simulink model "FishEyeTestNonCardboard_cs_old"  (R2018b)
settings: Solver=ode5  StartTime=0.0  StopTime=40  FixedStep=1/20  RelTol=1e-3
PreLoadFcn:
  | mbxruntime.callbacks.PreLoadFcn(bdroot);
PostLoadFcn:
  | mbxruntime.callbacks.PostLoadFcn(bdroot);
InitFcn:
  | mbxruntime.callbacks.InitFcn(bdroot);
StartFcn:
  | mbxruntime.callbacks.StartFcn(bdroot);
StopFcn:
  | mbxruntime.callbacks.StopFcn(bdroot);
model workspace (MAT data in the model file):
  mbox_table : struct (value not decoded)
  model_closed = 0
  sim_status = 0
undefined symbols (not defined in the file or in its folder): InitImageOutputDir
libraries: PreScanSimulinkLibrary x6, instrumentlib x1, simulink_extras x1
(part 1 of 2)
CloseFcn:
  | mbxruntime.callbacks.CloseFcn(bdroot);
settings Model: Creator=PRESCAN  LastModifiedBy=Kimoss
settings DataIOCC: LimitDataPoints=on  SaveFormat=Array  SignalLoggingSaveFormat=ModelDataLogs
settings OptimizationCC: ExpressionDepthLimit=2147483647  InitFltsAndDblsToZero=on  LifeSpan=inf
settings DebuggingCC: SaveWithParameterizedLinksMsg=none  UnderspecifiedInitializationDetection=Classic  MergeDetectMultiDrivingBlocksExec=none  SignalResolutionControl=TryResolveAllWithWarning  MultiTaskDSMMsg=warning  MultiTaskCondExecSysMsg=none  FcnCallInpInsideContextMsg=warning  StateNameClashWarn=warning  SFUnexpectedBacktrackingDiag=warning  SFNoUnconditionalDefaultTransitionDiag=warning  SFExecutionAtInitializationDiag=none
settings HardwareCC: ProdBitPerPointer=32  ProdBitPerSizeT=32  ProdBitPerPtrDiffT=32  ProdLargestAtomicFloat=None  ProdIntDivRoundTo=Undefined  ProdEndianess=Unspecified  ProdWordSize=32  ProdHWDeviceType=32-bit Generic
settings ModelReferenceCC: UpdateModelReferenceTargets=IfOutOfDate  PropagateSignalLabelsOutOfModel=off
settings SFSimCC: SimUseLocalCustomCode=off  SimParseCustomCode=off
settings SFSimCC: SimCustomHeaderCode=|
  | #include "prescan.h"
  | #include "prescan_platform.h"
settings RTWCC: RTWUseLocalCustomCode=off
settings CodeAppCC: StateflowObjectComments=on
settings GRTTargetCC: TargetFcnLib=ansi_tfl_tmw.mat  TargetLangStandard=C89/C90 (ANSI)  GeneratePreprocessorConditionals=Disable all  CombineOutputUpdateFcns=off  GRTInterface=on
settings ConfigComp: CovMetricSettings=dw  CovHtmlReporting=on  CovSaveCumulativeToWorkspaceVar=on  CovSaveSingleToWorkspaceVar=on  CovExternalEMLEnable=off

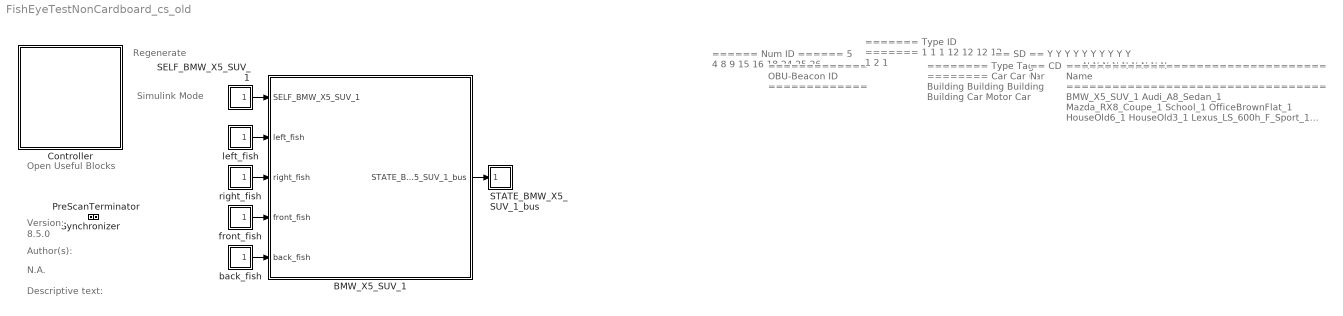
== system FishEyeTestNonCardboard_cs_old ==
  note: Regenerate
  note: Simulink Mode
  note: Open Useful Blocks
  note: 8.5.0
  note: Version:
  note: Author(s):
  note: N.A.
  note: Descriptive text:
  note: ======
      | Num ID
      | ======
      | 5
      | 4
      | 8
      | 9
      | 15
      | 16
      | 18
      | 24
      | 25
      | 26
  note: =============
      | OBU-Beacon ID
      | =============
  note: =======
      | Type ID
      | =======
      | 1
      | 1
      | 1
      | 12
      | 12
      | 12
      | 12
      | 1
      | 2
      | 1
  note: ========
      | Type Tag
      | ========
      | Car
      | Car
      | Car
      | Building
      | Building
      | Building
      | Building
      | Car
      | Motor
      | Car
  note: ==
      | SD
      | ==
      | Y
      | Y
      | Y
      | Y
      | Y
      | Y
      | Y
      | Y
      | Y
      | Y
  note: ==
      | CD
      | ==
      | N
      | N
      | N
      | N
      | N
      | N
      | N
      | N
      | N
      | N
  note: ==================================
      | Name
      | ==================================
      | BMW_X5_SUV_1
      | Audi_A8_Sedan_1
      | Mazda_RX8_Coupe_1
      | School_1
      | OfficeBrownFlat_1
      | HouseOld6_1
      | HouseOld3_1
      | Lexus_LS_600h_F_Sport_1
      | Honda_Pan_European_Motorcycle_With_Driver_1
      | Toyota_Previa_MPV_1
  BMW_X5_SUV_1 : Subsystem  Tag=WorldObjectSubSystem  InitFcn=UniqueId = '17';
      mask init:
      | modelPath = GenericModelHelper.getGenericModelFilePath('ModelDepo','Vehicles\BMW_X5\BMW_X5.pgmb','cea918691563e9ae3e6a88ec95e6726a');imagePath = GenericModelHelper.getCompilationPicture(modelPath, 'BMW_X5_HighPoly.png');
      mask Display: image(imread(imagePath));color('white');text(0, 0, ' ID=5\n')
  Controller : Subsystem  Description=F1E6339B9D6A8F6F92C51F5B65AEB1AE0C4158BDB2E3299F1705455A5C38CA89  Priority=-1  LoadFcn=load PreScanControllerData  mask(PreScan Simulation Controller){prescanversion='8.5.0', ModelReferencing=off, TimeStep=1/20, ControlMode=0, PreScanExecutionMode=on, ControllerCount=0, ControllerIndex=0, ControllerOptions=''}
      mask prompts: prescanversion "PreScan Version"; ModelReferencing "Use Model Referencing"; TimeStep "Upload Period [s]"; ControlMode "Control Mode"; PreScanExecutionMode "Execution Mode"; ControllerCount "Controller Count"; ControllerIndex "Controller Index"; ControllerOptions "Controller Options"
      mask help:
      | Please do not remove this block from the compilation sheet,
      | as it connects the model to the PreScan environment.
      mask init:
      | model = bdroot(gcb);
      | ExperimentFile = mbxruntime.findExperimentFile(model,true); %relative path
      | 
      | [d1, d2, d3, prescandata] = prescan_Settings();
      | ModelDepo = fullfile(prescandata,'ModelDepo'); 
      | 
      | RTmode = mbxruntime.getRTMode(model);
      | 
      | SimulationMode = get_param(bdroot,'SimulationMode');
      | if strcmp(SimulationMode, 'rapid-accelerator')
      |     SimulationMode = 'external';
      | end
      | TargetName = get_param(bdroot,'SystemTargetFile');
      settings: ModelCloseFcn=assignin('base',['model_closed_' bdroot],true);
      mask Help: eval('openHelp(812)')
      mask Display: image(imread('prescanlogo.ico'))
  PreScanTerminator : Subsystem  Tag=PreScanTerminator  Priority=999  LoadFcn=load PrescanTerminatorData  mask(PreScan Simulation Terminator){TimeStep=1/20}
      mask prompts: TimeStep "Upload Period [s]"
      mask help:
      | Please do not remove this block from the compilation sheet as it
      | connects the model to the PreScan environment.
      mask Help: eval('openHelp(812)')
      mask Display: image(imread('prescanlogo.ico'))
  SELF_BMW_X5_SUV_1 : Subsystem  Tag=sensor/SelfPort  Priority=3  LoadFcn=load('PreScanSelfSensorData.mat')  mask(PreScan Source Block: SELF){}
      mask help:
      | The SELF port shows (state) information of the actor itself. The outputs are position in the experiment's axis system and the GPS coordinates, and the object's absolute velocity and compass heading.
      |
      | For more information, please click Help.
      settings: OpenFcn=open_system([gcb '/Sensor'],'mask')
      mask Help: eval('openHelp(462)')
      mask Display: image(imread('GPS.png'))
  STATE_BMW_X5_SUV_1_bus : Subsystem  Tag=actuator/StatePort  Priority=0  LoadFcn=load('PreScanStateActuatorData.mat')  mask(PreScan Sink Block: State){}
      mask help:
      | The Actor State contains a vector signal of size (9x1), containing the following signals:
      |
      | -  Position    	(x,y,z)             	[m]
      | -  Velocity    	(vx,vy,vz)         	[m/s]
      | -  Angles       	(Roll, Pitch, Yaw)	[rad]
      |
      | The Actor state is defined in the global axis system.
      | The state is superponed on the Initial position defined in the GUI.
      |
      | For more information, please click Help.
      settings: OpenFcn=open_system([gcb '/Actuator'],'mask')
      mask Help: eval('openHelp(222)')
      mask Display: image(imread('State.png'))
  Synchronizer : Subsystem  Tag=PreScanSynchronizer  Priority=1  LoadFcn=load PrescanSynchronizeData  mask(PreScan Simulation Core Block){TimeStep=1/20}
      mask prompts: TimeStep "Timestep [s]"
      mask help:
      | Please do not remove this block from the PreScan compilation sheet,
      | as it contains essential configuration parameters for a PreScan simulation.
      settings: DeleteFcn=PreScanBlockDeleteFcn;
      mask Display: image(imread('prescanlogo.ico'))
  back_fish : Subsystem  Tag=sensor/Camera/FisheyeCamera  Priority=3  mask(PreScan Source Block: Fisheye Camera){}
      mask help: The Fisheye Camera provides a color or monochrome image.
      settings: OpenFcn=open_system([gcb '/Sensor'],'mask')
      mask Help: eval('openHelp(1461)')
      mask Display: image(imread('CameraSensor.png'))
  front_fish : Subsystem  Tag=sensor/Camera/FisheyeCamera  Priority=3  mask(PreScan Source Block: Fisheye Camera){}
      mask help: The Fisheye Camera provides a color or monochrome image.
      settings: OpenFcn=open_system([gcb '/Sensor'],'mask')
      mask Help: eval('openHelp(1461)')
      mask Display: image(imread('CameraSensor.png'))
  left_fish : Subsystem  Tag=sensor/Camera/FisheyeCamera  Priority=3  mask(PreScan Source Block: Fisheye Camera){}
      mask help: The Fisheye Camera provides a color or monochrome image.
      settings: OpenFcn=open_system([gcb '/Sensor'],'mask')
      mask Help: eval('openHelp(1461)')
      mask Display: image(imread('CameraSensor.png'))
  right_fish : Subsystem  Tag=sensor/Camera/FisheyeCamera  Priority=3  mask(PreScan Source Block: Fisheye Camera){}
      mask help: The Fisheye Camera provides a color or monochrome image.
      settings: OpenFcn=open_system([gcb '/Sensor'],'mask')
      mask Help: eval('openHelp(1461)')
      mask Display: image(imread('CameraSensor.png'))
  wires:
  BMW_X5_SUV_1/1(STATE_BMW_X5_SUV_1_bus) -> STATE_BMW_X5_SUV_1_bus/1(STATE_BMW_X5_SUV_1_bus)
  SELF_BMW_X5_SUV_1/1(SELF_BMW_X5_SUV_1) -> BMW_X5_SUV_1/1(SELF_BMW_X5_SUV_1)
  left_fish/1(left_fish) -> BMW_X5_SUV_1/2(left_fish)
  right_fish/1(right_fish) -> BMW_X5_SUV_1/3(right_fish)
  front_fish/1(front_fish) -> BMW_X5_SUV_1/4(front_fish)
  back_fish/1(back_fish) -> BMW_X5_SUV_1/5(back_fish)

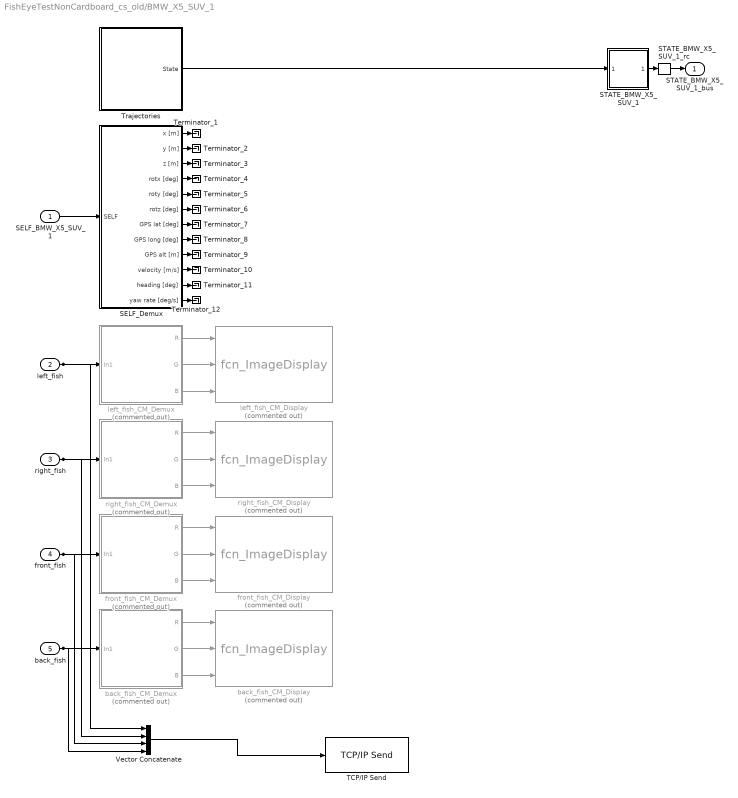
== system FishEyeTestNonCardboard_cs_old/BMW_X5_SUV_1 ==
  SELF_BMW_X5_SUV_1 : Inport  Tag=inport/SelfPort  OutDataTypeStr=Bus: PRESCAN_SELFSENSORDATA  PortDimensions=1  SampleTime=1/20  BusOutputAsStruct=on
  left_fish : Inport  Tag=inport/Camera/FisheyeCamera  Port=2  OutDataTypeStr=uint8  SampleTime=1/20  BusOutputAsStruct=on
  right_fish : Inport  Tag=inport/Camera/FisheyeCamera  Port=3  OutDataTypeStr=uint8  SampleTime=1/20  BusOutputAsStruct=on
  front_fish : Inport  Tag=inport/Camera/FisheyeCamera  Port=4  OutDataTypeStr=uint8  SampleTime=1/20  BusOutputAsStruct=on
  back_fish : Inport  Tag=inport/Camera/FisheyeCamera  Port=5  OutDataTypeStr=uint8  SampleTime=1/20  BusOutputAsStruct=on
  SELF_Demux : Subsystem  Tag=demux/SelfPort  mask(PreScan Demux Block:){}
      mask help:
      | The SELF port shows (state) information of the actor itself. The outputs are position in the experiment's axis system and the GPS coordinates, and the object's absolute velocity and compass heading.
      |
      | For more information, please click Help.
      settings: DeleteFcn=PreScanBlockDeleteFcn;
      mask Help: eval('openHelp(462)')
      mask Display:
      | port_label('output',1,'x [m]')
      | port_label('output',2,'y [m]')
      | port_label('output',3,'z [m]','texmode','on')
      | port_label('output',4,'Rotx [deg]','texmode','on')
      | port_label('output',5,'Roty [deg]','texmode','on')
      | port_label('output',6,'Rotz [deg]','texmode','on')
      | port_label('output',7,'GPS lat [deg]','texmode','on')
      | port_label('output',8,'GPS long [deg]','texmode','on')
      | port_label('output',9,'GPS alt [m]','texmode','on')
      | port_label('output',10,'Velocity [m/s]')
      | port_label('output',11,'Heading [deg]')
      | port_label('output',12,'Yaw rate [deg/s]')
  STATE_BMW_X5_SUV_1 : Subsystem  Tag=mux/StatePort  Priority=0  LoadFcn=load PrescanStateActuatorData  mask(PreScan Sink Block: State){x0=-88.414, y0=33.3612, z0=0.69, Roll0=0, Pitch0=0, Yaw0=360, TimeStep=1/20}
      mask prompts: x0 "Ini x-position VEHICLE wrt GLOBAL axis system [m]"; y0 "Ini y-position VEHICLE wrt GLOBAL axis system [m]"; z0 "Ini z-position VEHICLE wrt GLOBAL axis system [m]"; Roll0 "Ini roll-angle BODY wrt VEHICLE axis system [deg]"; Pitch0 "Ini pitch-angle BODY wrt VEHICLE axis system [deg]"; Yaw0 "Ini yaw-angle VEHICLE wrt GLOBAL axis system [deg]"; TimeStep "Auto-Assigned: Upload Period [s]"
      mask help:
      | The Actor State contains a vector signal of size (9x1), containing the following signals:
      |
      | -  Position                  (x,y,z)                                     [m]
      | -  Velocity                  (vx,vy,vz)                               [m/s]
      | -  Angles                    (Roll, Pitch, Yaw)                   [rad]
      |
      | The Actor state is defined in the global axis system.
      | The state is superponed on the Initial position defined in the GUI.
      |
      | For more information, please click Help.
      settings: DeleteFcn=PreScanBlockDeleteFcn;
      mask Help: eval('openHelp(222)')
      mask Display: image(imread('State.png'))
  STATE_BMW_X5_SUV_1_rc : RateTransition  Tag=mux_rc/StatePort  OutPortSampleTimeOpt=Inherit
  TCP/IP Send : instrumentlib/TCP//IP Send  Host=127.0.0.1  Port=1117  EnableBlockingMode=on  Timeout=10  ByteOrder=BigEndian  TransferDelay=on
      settings: SourceProductName=Instrument Control Toolbox
  Terminator_{1..12} (12 alike) : Terminator
  Trajectories : Subsystem  Tag=Trajectories  mask(PreScan Source Block: Trajectories){}
      mask help:
      | The Trajectory block contains the trajectories defined in the PreScan Experiment Editor. The output of the trajectory block is the (vehicle) State.
      |
      | For more information, please click Help.
      settings: DeleteFcn=PreScanBlockDeleteFcn;
      mask Help: eval('openHelp(312)')
      mask Display: image(imread('Trajectory.png'));
  Vector Concatenate : Concatenate  NumInputs=4  Mode=Multidimensional array  ConcatenateDimension=2
  back_fish_CM_Demux : Subsystem  Tag=demux/Camera/Color  Commented=on  mask{SensorName=back_fish, hres=640, vres=480}
      mask prompts: SensorName "Sensor Name"; hres "Horizontal Resolution"; vres "Vertical Resolution"
      mask Help: eval('openHelp(1461)')
      mask Display:
      | fprintf('MONO CAMERA:\n Color\n %s \n %d x %d px',SensorName,hres,vres)
      | port_label('output',1,'R')
      | port_label('output',2,'G')
      | port_label('output',3,'B')
  back_fish_CM_Display : M-S-Function  Tag=CameraSensor_Color_Display  Commented=on  InitFcn=InitImageOutputDir(gcb);  FunctionName=fcn_ImageDisplay  Parameters=SensorName EnableDisplay EnablePosition DisplayPosition FigureHandle SaveResults BitmapFormat TempOutputDir CameraType DataType  mask(PreScan Color Display Block){SensorName=back_fish, EnableDisplay=on, EnablePosition=off, DisplayPosition=[10 10 640 480], FigureHandle=1704, SaveResults=off, Format=PNG, TempOutputDir=0, CameraType=Mono, DataType=uint8}
      mask prompts: SensorName "User Specified: Title of Display"; EnableDisplay "Active"; EnablePosition "Set Display window position"; DisplayPosition "Display window position [xpos ypos width height]"; FigureHandle "Unique Handle"; SaveResults "Save results"; TempOutputDir "OutputDir"; CameraType "Camera Type"; DataType "Image Data Type"
      mask help: This block displays the RGB output of a PreScan camera sensor.
      mask init:
      | if EnableDisplay
      |     EnableString='';
      |     EnableColor='gray';
      | else
      |     EnableString='INACTIVE';
      |     EnableColor='red';
      | end
      | switch Format
      |     case 1
      |         BitmapFormat = 'png';
      |     case 2
      |         BitmapFormat = 'bmp';
      |     case 3
      |         BitmapFormat = 'jpg';
      | end 
      | if CameraType==1
      |     CameraTypeName='MONO';
      |     PortNumber=0;
      | else
      |     CameraTypeName='STEREO';
      |     PortNumber=3;
      | end
      settings: CopyFcn=CopyFcnDisplay  DeleteFcn=PreScanBlockDeleteFcn;  ModelCloseFcn=fcn_ImageDisplay_ModelCloseFcn
      mask Help: eval('openHelp(1461)')
      mask Callback EnablePosition:
      | MV=get_param(gcb,'MaskVisibilities');
      | if strcmp(get_param(gcb,'EnablePosition'),'on')
      |     MV{4}='on';
      | else
      |     MV{4}='off';
      | end
      | set_param(gcb,'MaskVisibilities',MV);
      | clear MV;
      mask TypeOptions Format: PNG | BMP | JPG
      mask TypeOptions CameraType: Mono | Stereo
      mask TypeOptions DataType: uint8 | single
      mask Display:
      | color(EnableColor);
      | fprintf('%s\n DISPLAY:\n Color \n %s',EnableString,SensorName)
      | port_label('input',1,'R')
      | port_label('input',2,'G')
      | port_label('input',3,'B')
      | port_label('input',PortNumber+1,'R')
      | port_label('input',PortNumber+2,'G')
      | port_label('input',PortNumber+3,'B')
  front_fish_CM_Demux : Subsystem  Tag=demux/Camera/Color  Commented=on  mask{SensorName=front_fish, hres=640, vres=480}
      mask prompts: SensorName "Sensor Name"; hres "Horizontal Resolution"; vres "Vertical Resolution"
      mask Help: eval('openHelp(1461)')
      mask Display:
      | fprintf('MONO CAMERA:\n Color\n %s \n %d x %d px',SensorName,hres,vres)
      | port_label('output',1,'R')
      | port_label('output',2,'G')
      | port_label('output',3,'B')
  front_fish_CM_Display : M-S-Function  Tag=CameraSensor_Color_Display  Commented=on  InitFcn=InitImageOutputDir(gcb);  FunctionName=fcn_ImageDisplay  Parameters=SensorName EnableDisplay EnablePosition DisplayPosition FigureHandle SaveResults BitmapFormat TempOutputDir CameraType DataType  mask(PreScan Color Display Block){SensorName=front_fish, EnableDisplay=on, EnablePosition=off, DisplayPosition=[10 10 640 480], FigureHandle=1703, SaveResults=off, Format=PNG, TempOutputDir=0, CameraType=Mono, DataType=uint8}
      mask prompts: SensorName "User Specified: Title of Display"; EnableDisplay "Active"; EnablePosition "Set Display window position"; DisplayPosition "Display window position [xpos ypos width height]"; FigureHandle "Unique Handle"; SaveResults "Save results"; TempOutputDir "OutputDir"; CameraType "Camera Type"; DataType "Image Data Type"
      mask help: This block displays the RGB output of a PreScan camera sensor.
      mask init: same as FishEyeTestNonCardboard_cs_old/BMW_X5_SUV_1/back_fish_CM_Display
      settings: CopyFcn=CopyFcnDisplay  DeleteFcn=PreScanBlockDeleteFcn;  ModelCloseFcn=fcn_ImageDisplay_ModelCloseFcn
      mask Help: eval('openHelp(1461)')
      mask Callback EnablePosition:
      | MV=get_param(gcb,'MaskVisibilities');
      | if strcmp(get_param(gcb,'EnablePosition'),'on')
      |     MV{4}='on';
      | else
      |     MV{4}='off';
      | end
      | set_param(gcb,'MaskVisibilities',MV);
      | clear MV;
      mask TypeOptions Format: PNG | BMP | JPG
      mask TypeOptions CameraType: Mono | Stereo
      mask TypeOptions DataType: uint8 | single
      mask Display:
      | color(EnableColor);
      | fprintf('%s\n DISPLAY:\n Color \n %s',EnableString,SensorName)
      | port_label('input',1,'R')
      | port_label('input',2,'G')
      | port_label('input',3,'B')
      | port_label('input',PortNumber+1,'R')
      | port_label('input',PortNumber+2,'G')
      | port_label('input',PortNumber+3,'B')
  left_fish_CM_Demux : Subsystem  Tag=demux/Camera/Color  Commented=on  mask{SensorName=left_fish, hres=640, vres=480}
      mask prompts: SensorName "Sensor Name"; hres "Horizontal Resolution"; vres "Vertical Resolution"
      mask Help: eval('openHelp(1461)')
      mask Display:
      | fprintf('MONO CAMERA:\n Color\n %s \n %d x %d px',SensorName,hres,vres)
      | port_label('output',1,'R')
      | port_label('output',2,'G')
      | port_label('output',3,'B')
  left_fish_CM_Display : M-S-Function  Tag=CameraSensor_Color_Display  Commented=on  InitFcn=InitImageOutputDir(gcb);  FunctionName=fcn_ImageDisplay  Parameters=SensorName EnableDisplay EnablePosition DisplayPosition FigureHandle SaveResults BitmapFormat TempOutputDir CameraType DataType  mask(PreScan Color Display Block){SensorName=left_fish, EnableDisplay=on, EnablePosition=off, DisplayPosition=[10 10 640 480], FigureHandle=1701, SaveResults=off, Format=PNG, TempOutputDir=0, CameraType=Mono, DataType=uint8}
      mask prompts: SensorName "User Specified: Title of Display"; EnableDisplay "Active"; EnablePosition "Set Display window position"; DisplayPosition "Display window position [xpos ypos width height]"; FigureHandle "Unique Handle"; SaveResults "Save results"; TempOutputDir "OutputDir"; CameraType "Camera Type"; DataType "Image Data Type"
      mask help: This block displays the RGB output of a PreScan camera sensor.
      mask init: same as FishEyeTestNonCardboard_cs_old/BMW_X5_SUV_1/back_fish_CM_Display
      settings: CopyFcn=CopyFcnDisplay  DeleteFcn=PreScanBlockDeleteFcn;  ModelCloseFcn=fcn_ImageDisplay_ModelCloseFcn
      mask Help: eval('openHelp(1461)')
      mask Callback EnablePosition:
      | MV=get_param(gcb,'MaskVisibilities');
      | if strcmp(get_param(gcb,'EnablePosition'),'on')
      |     MV{4}='on';
      | else
      |     MV{4}='off';
      | end
      | set_param(gcb,'MaskVisibilities',MV);
      | clear MV;
      mask TypeOptions Format: PNG | BMP | JPG
      mask TypeOptions CameraType: Mono | Stereo
      mask TypeOptions DataType: uint8 | single
      mask Display:
      | color(EnableColor);
      | fprintf('%s\n DISPLAY:\n Color \n %s',EnableString,SensorName)
      | port_label('input',1,'R')
      | port_label('input',2,'G')
      | port_label('input',3,'B')
      | port_label('input',PortNumber+1,'R')
      | port_label('input',PortNumber+2,'G')
      | port_label('input',PortNumber+3,'B')
  right_fish_CM_Demux : Subsystem  Tag=demux/Camera/Color  Commented=on  mask{SensorName=right_fish, hres=640, vres=480}
      mask prompts: SensorName "Sensor Name"; hres "Horizontal Resolution"; vres "Vertical Resolution"
      mask Help: eval('openHelp(1461)')
      mask Display:
      | fprintf('MONO CAMERA:\n Color\n %s \n %d x %d px',SensorName,hres,vres)
      | port_label('output',1,'R')
      | port_label('output',2,'G')
      | port_label('output',3,'B')
  right_fish_CM_Display : M-S-Function  Tag=CameraSensor_Color_Display  Commented=on  InitFcn=InitImageOutputDir(gcb);  FunctionName=fcn_ImageDisplay  Parameters=SensorName EnableDisplay EnablePosition DisplayPosition FigureHandle SaveResults BitmapFormat TempOutputDir CameraType DataType  mask(PreScan Color Display Block){SensorName=right_fish, EnableDisplay=on, EnablePosition=off, DisplayPosition=[10 10 640 480], FigureHandle=1702, SaveResults=off, Format=PNG, TempOutputDir=0, CameraType=Mono, DataType=uint8}
      mask prompts: SensorName "User Specified: Title of Display"; EnableDisplay "Active"; EnablePosition "Set Display window position"; DisplayPosition "Display window position [xpos ypos width height]"; FigureHandle "Unique Handle"; SaveResults "Save results"; TempOutputDir "OutputDir"; CameraType "Camera Type"; DataType "Image Data Type"
      mask help: This block displays the RGB output of a PreScan camera sensor.
      mask init: same as FishEyeTestNonCardboard_cs_old/BMW_X5_SUV_1/back_fish_CM_Display
      settings: CopyFcn=CopyFcnDisplay  DeleteFcn=PreScanBlockDeleteFcn;  ModelCloseFcn=fcn_ImageDisplay_ModelCloseFcn
      mask Help: eval('openHelp(1461)')
      mask Callback EnablePosition:
      | MV=get_param(gcb,'MaskVisibilities');
      | if strcmp(get_param(gcb,'EnablePosition'),'on')
      |     MV{4}='on';
      | else
      |     MV{4}='off';
      | end
      | set_param(gcb,'MaskVisibilities',MV);
      | clear MV;
      mask TypeOptions Format: PNG | BMP | JPG
      mask TypeOptions CameraType: Mono | Stereo
      mask TypeOptions DataType: uint8 | single
      mask Display:
      | color(EnableColor);
      | fprintf('%s\n DISPLAY:\n Color \n %s',EnableString,SensorName)
      | port_label('input',1,'R')
      | port_label('input',2,'G')
      | port_label('input',3,'B')
      | port_label('input',PortNumber+1,'R')
      | port_label('input',PortNumber+2,'G')
      | port_label('input',PortNumber+3,'B')
  STATE_BMW_X5_SUV_1_bus : Outport  Tag=outport/StatePort  OutDataTypeStr=Bus: PRESCAN_STATEACTUATORDATA  PortDimensions=1  SampleTime=1/20
  wires:
  left_fish/1 -> Vector Concatenate/1, left_fish_CM_Demux/1(In1)
  right_fish/1 -> Vector Concatenate/2, right_fish_CM_Demux/1(In1)
  front_fish/1 -> Vector Concatenate/3, front_fish_CM_Demux/1(In1)
  back_fish/1 -> Vector Concatenate/4, back_fish_CM_Demux/1(In1)
  Vector Concatenate/1 -> TCP/IP Send/1
  STATE_BMW_X5_SUV_1_rc/1 -> STATE_BMW_X5_SUV_1_bus/1
  STATE_BMW_X5_SUV_1/1(StateBus) -> STATE_BMW_X5_SUV_1_rc/1
  SELF_BMW_X5_SUV_1/1 -> SELF_Demux/1(SELF)
  left_fish_CM_Demux/1(R) -> left_fish_CM_Display/1
  left_fish_CM_Demux/2(G) -> left_fish_CM_Display/2
  left_fish_CM_Demux/3(B) -> left_fish_CM_Display/3
  right_fish_CM_Demux/1(R) -> right_fish_CM_Display/1
  right_fish_CM_Demux/2(G) -> right_fish_CM_Display/2
  right_fish_CM_Demux/3(B) -> right_fish_CM_Display/3
  front_fish_CM_Demux/1(R) -> front_fish_CM_Display/1
  front_fish_CM_Demux/2(G) -> front_fish_CM_Display/2
  front_fish_CM_Demux/3(B) -> front_fish_CM_Display/3
  back_fish_CM_Demux/1(R) -> back_fish_CM_Display/1
  back_fish_CM_Demux/2(G) -> back_fish_CM_Display/2
  back_fish_CM_Demux/3(B) -> back_fish_CM_Display/3
  Trajectories/1(State) -> STATE_BMW_X5_SUV_1/1(State)
  SELF_Demux/1(x [m]) -> Terminator_1/1
  SELF_Demux/2(y [m]) -> Terminator_2/1
  SELF_Demux/3(z [m]) -> Terminator_3/1
  SELF_Demux/4(rotx [deg]) -> Terminator_4/1
  SELF_Demux/5(roty [deg]) -> Terminator_5/1
  SELF_Demux/6(rotz [deg]) -> Terminator_6/1
  SELF_Demux/7(GPS lat [deg]) -> Terminator_7/1
  SELF_Demux/8(GPS long [deg]) -> Terminator_8/1
  SELF_Demux/9(GPS alt [m]) -> Terminator_9/1
  SELF_Demux/10(velocity [m/s]) -> Terminator_10/1
  SELF_Demux/11(heading [deg]) -> Terminator_11/1
  SELF_Demux/12(yaw rate [deg/s]) -> Terminator_12/1

== system FishEyeTestNonCardboard_cs_old/Controller ==
  Terminator : Terminator
  sfun_Controller : S-Function  FunctionName=sfun_Controller  Parameters=SParameter1, SParameter2, SParameter3, SParameter4, SParameter5, SParameter6, SParameter7, SParameter8, SParameter9, SParameter10, SampleTime  SFunctionDeploymentMode=off  EnableBusSupport=off  mask(Legacy Function){SFunctionSpec=void prescan_outputFcn(void** work1, PRESCAN_CONTROLLERDATA y1[1]), SParameter1=uint8([ExperimentFile 0]), SParameter2=uint8([ModelDepo 0]), SParameter3=uint8([ControllerOptions 0]), SParameter4=RTmode, SParameter5=PreScanExecutionMode, SParameter6=ControlMode, SParameter7=ControllerCount, SParameter8=ControllerIndex, SParameter9=uint8([SimulationMode 0]), SParameter10=uint8([TargetName 0]), SampleTime=TimeStep, ShowSpec=on}
      mask prompts: SParameter1 "P1:"; SParameter2 "P2:"; SParameter3 "P3:"; SParameter4 "P4:"; SParameter5 "P5:"; SParameter6 "P6:"; SParameter7 "P7:"; SParameter8 "P8:"; SParameter9 "P9:"; SParameter10 "P10:"; SampleTime "Sample time (-1 for inherited):"; ShowSpec "Display function specification"
      mask help:
      | This block allows you to call the legacy functions specified by the following Legacy Code Tool definition:
      | def.SFunctionName = 'sfun_Controller';
      | def.OutputFcnSpec = 'void prescan_outputFcn(void** work1, PRESCAN_CONTROLLERDATA y1[1])';
      | def.StartFcnSpec = 'void prescan_startFcn(void ** work1, uint8 p1[], uint8 p2[], uint8 p3[], double p4, double p5, double p6, double p7, double p8, uint8 p9[], uint8 p10[])';
      | def.TerminateFcnSpec = 'void prescan_terminateFcn(void** work1)';
      | def.HeaderFiles = {'prescan_controller_data.h', 'prescan_SFunLibrary.h', 'prescan_CreateLogHandler.h', 'prescan_CreateErrorHandler.h', 'prescan_modify.h', 'ModuleDLL.h'};
      | def.SourceFiles = {'prescan_MexLogHandler.c', 'prescan_SimStructErrorHandler.c', 'prescan_LogHandler.c', 'prescan_ErrorHandler.c', 'prescan_Modify.c'};
      | def.HostLibFiles = {'sensorinterfaced.lib'};
      | def.TargetLibFiles = {'sensorinterfaced.so'};
      | def.IncPaths = {'.', 'C:\projects\prescan\rt_vislibrary\vis\..\pimp\include\sensors\InterfaceRTW'};
      | def.SrcPaths = {'C:\projects\prescan\rt_vislibrary\vis\..\pimp\include\sensors\InterfaceRTW', 'C:\projects\prescan\rt_vislibrary\vis\..\pimp\include\sensors\InterfaceRTW\ccurrt'};
      | def.LibPaths = {'C:\\projects\\prescan\\vislibrary_build\lib'};
      | def.SampleTime = 'parameterized';
      mask Help: <p>This block was generated automatically by the Legacy Code Tool. For detailed help on this tool, call<a href="matlab:legacy_code('help')"> legacy_code('help')</a>.</p>
      mask Callback ShowSpec:
      | if strcmp(get_param(gcbh, 'ShowSpec'), 'on')
      |   set_param(gcbh, 'MaskDisplay', sprintf('fprintf(''%s'');', get_param(gcbh, 'SFunctionSpec')));
      | else
      |   set_param(gcbh, 'MaskDisplay', sprintf('fprintf(''%s'');', get_param(gcbh, 'FunctionName')));
      | end
      mask Display: fprintf('void prescan_outputFcn(void** work1, PRESCAN_CONTROLLERDATA y1[1])');
  wires:
  sfun_Controller/1 -> Terminator/1

== system FishEyeTestNonCardboard_cs_old/PreScanTerminator ==
  Terminator : Terminator
  sfun_Terminator : S-Function  FunctionName=sfun_Terminator  Parameters=SampleTime  SFunctionDeploymentMode=off  EnableBusSupport=off  mask(Legacy Function){SFunctionSpec=void prescan_terminator_outputFcn(void ** work1, PRESCAN_TERMINATORDATA y1[1]), SampleTime=TimeStep, ShowSpec=on}
      mask prompts: SampleTime "Sample time (-1 for inherited):"; ShowSpec "Display function specification"
      mask help:
      | This block allows you to call the legacy functions specified by the following Legacy Code Tool definition:
      | def.SFunctionName = 'sfun_Terminator';
      | def.OutputFcnSpec = 'void prescan_terminator_outputFcn(void ** work1, PRESCAN_TERMINATORDATA y1[1])';
      | def.StartFcnSpec = 'void prescan_terminator_startFcn(void ** work1)';
      | def.TerminateFcnSpec = 'void prescan_terminator_terminateFcn(void ** work1)';
      | def.HeaderFiles = {'prescan_terminator_data.h'};
      | def.HostLibFiles = {'sensorinterfaced.lib'};
      | def.IncPaths = {'src', 'C:\prescandev\vislibrary\vis\..\pimp\include\sensors\InterfaceRTW'};
      | def.SrcPaths = {'src'};
      | def.LibPaths = {'C:\\prescandev\\vislibrary_build\lib'};
      | def.SampleTime = 'parameterized';
      | def.Options.language = 'C';
      mask Help: <p>This block was generated automatically by the Legacy Code Tool. For detailed help on this tool, call<a href="matlab:legacy_code('help')"> legacy_code('help')</a>.</p>
      mask Callback ShowSpec:
      | if strcmp(get_param(gcbh, 'ShowSpec'), 'on')
      |   set_param(gcbh, 'MaskDisplay', sprintf('fprintf(''%s'');', get_param(gcbh, 'SFunctionSpec')));
      | else
      |   set_param(gcbh, 'MaskDisplay', sprintf('fprintf(''%s'');', get_param(gcbh, 'FunctionName')));
      | end
      mask Display: fprintf('void prescan_terminator_outputFcn(void ** work1, PRESCAN_TERMINATORDATA y1[1])');
  wires:
  sfun_Terminator/1 -> Terminator/1

== system FishEyeTestNonCardboard_cs_old/SELF_BMW_X5_SUV_1 ==
  Sensor : S-Function  FunctionName=sfun_SelfSensor  Parameters=UniqueID, TimeStep  SFunctionDeploymentMode=off  EnableBusSupport=off  mask(PreScan Source Block: SELF){UniqueID=17, TimeStep=1/20}
      mask prompts: UniqueID "Auto-Assigned: Unique ID"; TimeStep "Auto-Assigned: Upload Period [s]"
      mask help:
      | The SELF port shows (state) information of the actor itself. The outputs are position in the experiment's axis system and the GPS coordinates, and the object's absolute velocity and compass heading.
      |
      | For more information, please click Help.
      mask Help: eval('openHelp(462)')
      mask Display: image(imread('GPS.png'))
  SELF_BMW_X5_SUV_1 : Outport  Tag=outport/SelfPort  OutDataTypeStr=Bus: PRESCAN_SELFSENSORDATA  PortDimensions=1  SampleTime=1/20
  wires:
  Sensor/1 -> SELF_BMW_X5_SUV_1/1

== system FishEyeTestNonCardboard_cs_old/STATE_BMW_X5_SUV_1_bus ==
  STATE_BMW_X5_SUV_1_bus : Inport  Tag=inport/StatePort  OutDataTypeStr=Bus: PRESCAN_STATEACTUATORDATA  PortDimensions=1  SampleTime=1/20  BusOutputAsStruct=on
  Actuator : S-Function  FunctionName=sfun_StateActuator  Parameters=UniqueID, TimeStep  SFunctionDeploymentMode=off  EnableBusSupport=off  mask(PreScan Sink Block: State){UniqueID=17, TimeStep=1/20}
      mask prompts: UniqueID "Auto-Assigned: Unique ID"; TimeStep "Auto-Assigned: Upload Period [s]"
      mask help:
      | The Actor State contains a vector signal of size (9x1), containing the following signals:
      |
      | -  Position    	(x,y,z)             	[m]
      | -  Velocity    	(vx,vy,vz)         	[m/s]
      | -  Angles       	(Roll, Pitch, Yaw)	[rad]
      |
      | The Actor state is defined in the global axis system.
      | The state is superponed on the Initial position defined in the GUI.
      |
      | For more information, please click Help.
      mask Help: eval('openHelp(222)')
      mask Display: image(imread('State.png'))
  wires:
  STATE_BMW_X5_SUV_1_bus/1 -> Actuator/1

== system FishEyeTestNonCardboard_cs_old/Synchronizer ==
  Bus Selector1 : BusSelector  OutputSignals=FederateStopped
  Stop Simulation : Stop
  sfun_Synchronizer : S-Function  FunctionName=sfun_Synchronizer  Parameters=SampleTime  SFunctionDeploymentMode=off  EnableBusSupport=off  mask(Legacy Function){SFunctionSpec=void prescan_synchronizer_outputFcn(void ** work1, PRESCAN_SYNCHRONIZEDATA y1[1]), SampleTime=TimeStep, ShowSpec=on}
      mask prompts: SampleTime "Sample time (-1 for inherited):"; ShowSpec "Display function specification"
      mask help:
      | This block allows you to call the legacy functions specified by the following Legacy Code Tool definition:
      | def.SFunctionName = 'sfun_Synchronizer';
      | def.OutputFcnSpec = 'void prescan_synchronizer_outputFcn(void ** work1, PRESCAN_SYNCHRONIZEDATA y1[1])';
      | def.StartFcnSpec = 'void prescan_synchronizer_startFcn(void ** work1)';
      | def.TerminateFcnSpec = 'void prescan_synchronizer_terminateFcn(void ** work1)';
      | def.HeaderFiles = {'prescan_synchronizer_data.h'};
      | def.HostLibFiles = {'sensorinterfaced.lib'};
      | def.IncPaths = {'src', 'C:\prescandev\vislibrary\vis\..\pimp\include\sensors\InterfaceRTW'};
      | def.SrcPaths = {'src'};
      | def.LibPaths = {'C:\\prescandev\\vislibrary_build\lib'};
      | def.SampleTime = 'parameterized';
      | def.Options.language = 'C';
      mask Help: <p>This block was generated automatically by the Legacy Code Tool. For detailed help on this tool, call<a href="matlab:legacy_code('help')"> legacy_code('help')</a>.</p>
      mask Callback ShowSpec:
      | if strcmp(get_param(gcbh, 'ShowSpec'), 'on')
      |   set_param(gcbh, 'MaskDisplay', sprintf('fprintf(''%s'');', get_param(gcbh, 'SFunctionSpec')));
      | else
      |   set_param(gcbh, 'MaskDisplay', sprintf('fprintf(''%s'');', get_param(gcbh, 'FunctionName')));
      | end
      mask Display: fprintf('void prescan_synchronizer_outputFcn(void ** work1, PRESCAN_SYNCHRONIZEDATA y1[1])');
  wires:
  Bus Selector1/1 -> Stop Simulation/1  "<FederateStopped>"
  sfun_Synchronizer/1 -> Bus Selector1/1

== system FishEyeTestNonCardboard_cs_old/back_fish ==
  Sensor : S-Function  FunctionName=sfun_Camera  Parameters=sensorID, dataWidth, dataHeight, channelsPerImage, numberOfImages, timestep  SFunctionDeploymentMode=off  EnableBusSupport=off  mask(PreScan Source Block: Fisheye Camera){sensorID=31, dataWidth=480, dataHeight=1920, channelsPerImage=3, numberOfImages=1, timestep=1/20}
      mask prompts: sensorID "Sensor ID"; dataWidth "Data width"; dataHeight "Data Height"; channelsPerImage "Channels per image"; numberOfImages "Number of images"; timestep "MATLAB timestep:"
      mask help: The Fisheye Camera provides a color or monochrome image.
      mask Help: eval('openHelp(1461)')
      mask Display: image(imread('CameraSensor.png'))
  back_fish : Outport  Tag=outport/Camera/FisheyeCamera  OutDataTypeStr=uint8  SampleTime=1/20
  wires:
  Sensor/1 -> back_fish/1

== system FishEyeTestNonCardboard_cs_old/front_fish ==
  Sensor : S-Function  FunctionName=sfun_Camera  Parameters=sensorID, dataWidth, dataHeight, channelsPerImage, numberOfImages, timestep  SFunctionDeploymentMode=off  EnableBusSupport=off  mask(PreScan Source Block: Fisheye Camera){sensorID=29, dataWidth=480, dataHeight=1920, channelsPerImage=3, numberOfImages=1, timestep=1/20}
      mask prompts: sensorID "Sensor ID"; dataWidth "Data width"; dataHeight "Data Height"; channelsPerImage "Channels per image"; numberOfImages "Number of images"; timestep "MATLAB timestep:"
      mask help: The Fisheye Camera provides a color or monochrome image.
      mask Help: eval('openHelp(1461)')
      mask Display: image(imread('CameraSensor.png'))
  front_fish : Outport  Tag=outport/Camera/FisheyeCamera  OutDataTypeStr=uint8  SampleTime=1/20
  wires:
  Sensor/1 -> front_fish/1

== system FishEyeTestNonCardboard_cs_old/left_fish ==
  Sensor : S-Function  FunctionName=sfun_Camera  Parameters=sensorID, dataWidth, dataHeight, channelsPerImage, numberOfImages, timestep  SFunctionDeploymentMode=off  EnableBusSupport=off  mask(PreScan Source Block: Fisheye Camera){sensorID=18, dataWidth=480, dataHeight=1920, channelsPerImage=3, numberOfImages=1, timestep=1/20}
      mask prompts: sensorID "Sensor ID"; dataWidth "Data width"; dataHeight "Data Height"; channelsPerImage "Channels per image"; numberOfImages "Number of images"; timestep "MATLAB timestep:"
      mask help: The Fisheye Camera provides a color or monochrome image.
      mask Help: eval('openHelp(1461)')
      mask Display: image(imread('CameraSensor.png'))
  left_fish : Outport  Tag=outport/Camera/FisheyeCamera  OutDataTypeStr=uint8  SampleTime=1/20
  wires:
  Sensor/1 -> left_fish/1

== system FishEyeTestNonCardboard_cs_old/right_fish ==
  Sensor : S-Function  FunctionName=sfun_Camera  Parameters=sensorID, dataWidth, dataHeight, channelsPerImage, numberOfImages, timestep  SFunctionDeploymentMode=off  EnableBusSupport=off  mask(PreScan Source Block: Fisheye Camera){sensorID=28, dataWidth=480, dataHeight=1920, channelsPerImage=3, numberOfImages=1, timestep=1/20}
      mask prompts: sensorID "Sensor ID"; dataWidth "Data width"; dataHeight "Data Height"; channelsPerImage "Channels per image"; numberOfImages "Number of images"; timestep "MATLAB timestep:"
      mask help: The Fisheye Camera provides a color or monochrome image.
      mask Help: eval('openHelp(1461)')
      mask Display: image(imread('CameraSensor.png'))
  right_fish : Outport  Tag=outport/Camera/FisheyeCamera  OutDataTypeStr=uint8  SampleTime=1/20
  wires:
  Sensor/1 -> right_fish/1

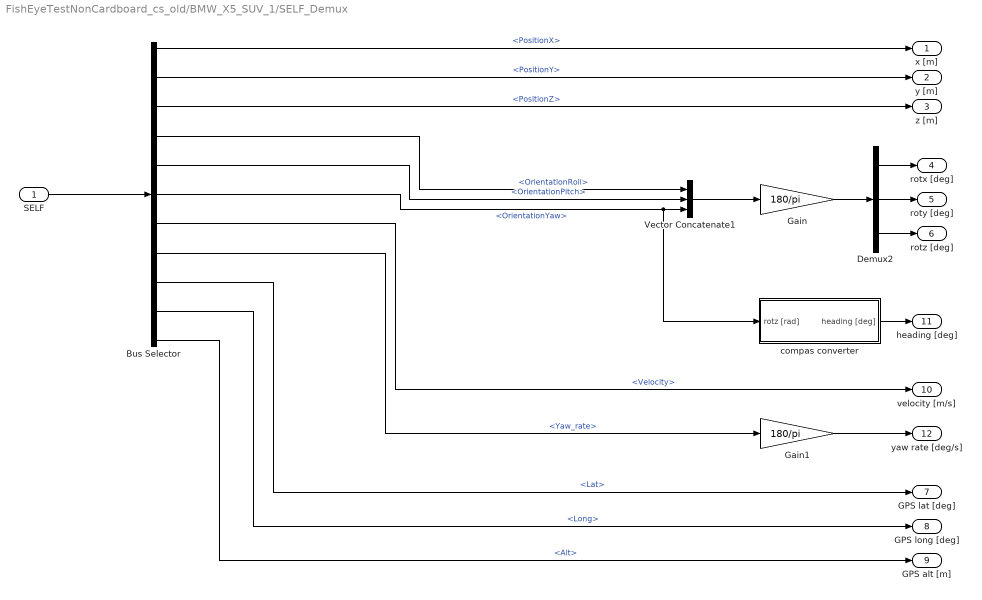
== system FishEyeTestNonCardboard_cs_old/BMW_X5_SUV_1/SELF_Demux ==
  SELF : Inport  OutDataTypeStr=Bus: PRESCAN_SELFSENSORDATA
  Bus Selector : BusSelector  OutputSignals=PositionX,PositionY,PositionZ,OrientationRoll,OrientationPitch,OrientationYaw,Velocity,Yaw_rate,Lat,Long,Alt
  Demux2 : Demux  Outputs=3
  Gain : Gain  Gain=180/pi
  Gain1 : Gain  Gain=180/pi
  Vector Concatenate1 : Concatenate  NumInputs=3
  compas converter : Subsystem
  x [m] : Outport
  y [m] : Outport  Port=2
  z [m] : Outport  Port=3
  rotx [deg] : Outport  Port=4
  roty [deg] : Outport  Port=5
  rotz [deg] : Outport  Port=6
  GPS lat [deg] : Outport  Port=7
  GPS long [deg] : Outport  Port=8
  GPS alt [m] : Outport  Port=9
  velocity [m/s] : Outport  Port=10
  heading [deg] : Outport  Port=11
  yaw rate [deg/s] : Outport  Port=12
  wires:
  Bus Selector/11 -> GPS alt [m]/1  "<Alt>"
  Bus Selector/10 -> GPS long [deg]/1  "<Long>"
  Bus Selector/9 -> GPS lat [deg]/1  "<Lat>"
  Bus Selector/8 -> Gain1/1  "<Yaw_rate>"
  Bus Selector/7 -> velocity [m/s]/1  "<Velocity>"
  Bus Selector/6 -> compas converter/1(rotz [rad]), Vector Concatenate1/3  "<OrientationYaw>"
  Bus Selector/5 -> Vector Concatenate1/2  "<OrientationPitch>"
  Bus Selector/4 -> Vector Concatenate1/1  "<OrientationRoll>"
  Vector Concatenate1/1 -> Gain/1
  Bus Selector/3 -> z [m]/1  "<PositionZ>"
  Bus Selector/2 -> y [m]/1  "<PositionY>"
  Bus Selector/1 -> x [m]/1  "<PositionX>"
  SELF/1 -> Bus Selector/1
  Gain/1 -> Demux2/1
  Demux2/1 -> rotx [deg]/1
  Demux2/2 -> roty [deg]/1
  Demux2/3 -> rotz [deg]/1
  compas converter/1(heading [deg]) -> heading [deg]/1
  Gain1/1 -> yaw rate [deg/s]/1

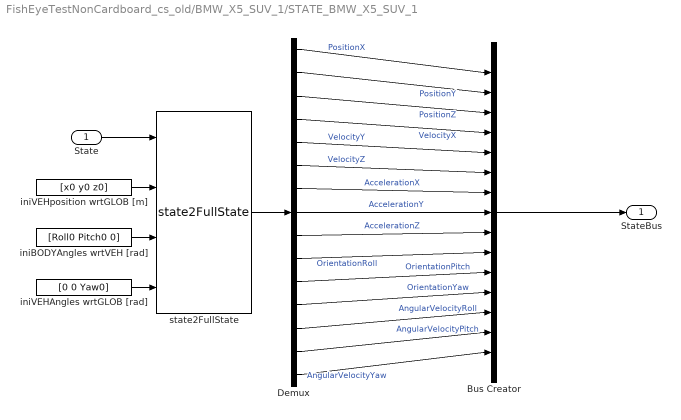
== system FishEyeTestNonCardboard_cs_old/BMW_X5_SUV_1/STATE_BMW_X5_SUV_1 ==
  State : Inport  SampleTime=TimeStep
  Bus Creator : BusCreator  Inputs=15  OutDataTypeStr=Bus: PRESCAN_STATEACTUATORDATA  NonVirtualBus=on
  Demux : Demux  Outputs=15
  iniBODYAngles wrtVEH [rad] : Constant  Value=[Roll0 Pitch0 0]  SampleTime=TimeStep
  iniVEHAngles wrtGLOB [rad] : Constant  Value=[0 0 Yaw0]  SampleTime=TimeStep
  iniVEHposition wrtGLOB [m] : Constant  Value=[x0 y0 z0]  SampleTime=TimeStep
  state2FullState : PreScanSimulinkLibrary/state2FullState  SystemSampleTime=-1
  StateBus : Outport  OutDataTypeStr=Bus: PRESCAN_STATEACTUATORDATA
  wires:
  Bus Creator/1 -> StateBus/1
  State/1 -> state2FullState/1
  state2FullState/1 -> Demux/1
  iniVEHposition wrtGLOB [m]/1 -> state2FullState/2
  iniBODYAngles wrtVEH [rad]/1 -> state2FullState/3
  iniVEHAngles wrtGLOB [rad]/1 -> state2FullState/4
  Demux/1 -> Bus Creator/1  "PositionX"
  Demux/2 -> Bus Creator/2  "PositionY"
  Demux/3 -> Bus Creator/3  "PositionZ"
  Demux/4 -> Bus Creator/4  "VelocityX"
  Demux/5 -> Bus Creator/5  "VelocityY"
  Demux/6 -> Bus Creator/6  "VelocityZ"
  Demux/7 -> Bus Creator/7  "AccelerationX"
  Demux/8 -> Bus Creator/8  "AccelerationY"
  Demux/9 -> Bus Creator/9  "AccelerationZ"
  Demux/10 -> Bus Creator/10  "OrientationRoll"
  Demux/11 -> Bus Creator/11  "OrientationPitch"
  Demux/12 -> Bus Creator/12  "OrientationYaw"
  Demux/13 -> Bus Creator/13  "AngularVelocityRoll"
  Demux/14 -> Bus Creator/14  "AngularVelocityPitch"
  Demux/15 -> Bus Creator/15  "AngularVelocityYaw"

== system FishEyeTestNonCardboard_cs_old/BMW_X5_SUV_1/Trajectories ==
  Traj2State1 : Subsystem  Tag=Traj2State  mask(PreScan Demux Block:){}
      settings: DeleteFcn=PreScanBlockDeleteFcn;
  TrajCoGOffset : Subsystem  Tag=TrajCoGOffset  mask(Trajectory CoG Offset block){CoGOffsetZ=0.69, InitRoll=0, InitPitch=0}
      mask prompts: CoGOffsetZ "Z-component of CoG Offset [m]:"; InitRoll "Initial Roll angle [deg]:"; InitPitch "Initial Pitch angle [deg]:"
      mask help: A trajectory follows the surface of the road. However the position of a actor is based on the actor's Center of Gravity, which is typically above the road. This block converts from the trajectory along the road surface to the trajectory of the actor's CoG by realigning the z-component of the CoG offset to be normal to the road.
      settings: DeleteFcn=PreScanBlockDeleteFcn;
  Trajectory_1 : Subsystem  Tag=Trajectory  mask(PreScan Source Block: Trajectory){FileName='Trajectory_1.mat', TimeStep=1/20}
      mask prompts: TimeStep "Time Step [s]"
      mask help:
      | The Trajectory block contains the trajectories defined in the PreScan Experiment Editor. The output of the trajectory block is the (vehicle) State.
      |
      | For more information, please click Help.
      mask init:
      | EXPROOT=pwd;  % TODO better construction for locating base experiment
      | 
      | trajfilename = fullfile(EXPROOT,'Trajectories',FileName);
      | load(trajfilename);
      | trajectory=trajectory';
      | 
      | traj.time=trajectory(:,1);%[];
      | traj.signals.values=trajectory(:,2:19);
      | traj.dimensions=18;
      | traj.label='';
      | 
      | SampleTime=traj.time(2)-traj.time(1);
      settings: DeleteFcn=PreScanBlockDeleteFcn;
      mask Help: eval('openHelp(312)')
      mask Display: fprintf(FileName)
  Trajectory_1_Offset : Constant  Tag=TrajectoryOffset  Value="[0  0  0  0  0  0]"
  State : Outport  Tag=TrajOutport
  wires:
  Trajectory_1/1(trajectory) -> Traj2State1/1(Traj Org)
  Trajectory_1_Offset/1 -> Traj2State1/2(Offset)
  TrajCoGOffset/1(State Out) -> State/1
  Traj2State1/1(state) -> TrajCoGOffset/1(State In)

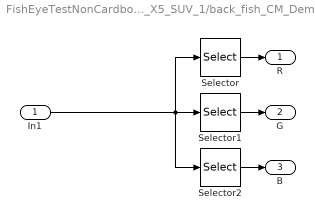
== system FishEyeTestNonCardboard_cs_old/BMW_X5_SUV_1/back_fish_CM_Demux ==
  In1 : Inport
  Selector : Selector  NumberOfDimensions=2  InputPortWidth=3  IndexOptions=Index vector (dialog),Index vector (dialog)  Indices=-1,1:hres  OutputSizes=1,1
  Selector1 : Selector  NumberOfDimensions=2  InputPortWidth=3  IndexOptions=Index vector (dialog),Index vector (dialog)  Indices=-1,hres+1:hres*2  OutputSizes=1,1
  Selector2 : Selector  NumberOfDimensions=2  InputPortWidth=3  IndexOptions=Index vector (dialog),Index vector (dialog)  Indices=-1,hres*2+1:hres*3  OutputSizes=1,1
  R : Outport
  G : Outport  Port=2
  B : Outport  Port=3
  wires:
  In1/1 -> Selector1/1, Selector/1, Selector2/1
  Selector/1 -> R/1
  Selector1/1 -> G/1
  Selector2/1 -> B/1

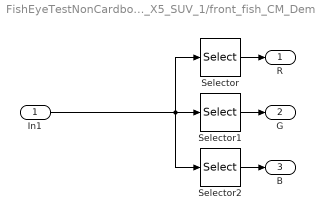
== system FishEyeTestNonCardboard_cs_old/BMW_X5_SUV_1/front_fish_CM_Demux ==
  In1 : Inport
  Selector : Selector  NumberOfDimensions=2  InputPortWidth=3  IndexOptions=Index vector (dialog),Index vector (dialog)  Indices=-1,1:hres  OutputSizes=1,1
  Selector1 : Selector  NumberOfDimensions=2  InputPortWidth=3  IndexOptions=Index vector (dialog),Index vector (dialog)  Indices=-1,hres+1:hres*2  OutputSizes=1,1
  Selector2 : Selector  NumberOfDimensions=2  InputPortWidth=3  IndexOptions=Index vector (dialog),Index vector (dialog)  Indices=-1,hres*2+1:hres*3  OutputSizes=1,1
  R : Outport
  G : Outport  Port=2
  B : Outport  Port=3
  wires:
  In1/1 -> Selector1/1, Selector/1, Selector2/1
  Selector/1 -> R/1
  Selector1/1 -> G/1
  Selector2/1 -> B/1

== system FishEyeTestNonCardboard_cs_old/BMW_X5_SUV_1/left_fish_CM_Demux ==
  In1 : Inport
  Selector : Selector  NumberOfDimensions=2  InputPortWidth=3  IndexOptions=Index vector (dialog),Index vector (dialog)  Indices=-1,1:hres  OutputSizes=1,1
  Selector1 : Selector  NumberOfDimensions=2  InputPortWidth=3  IndexOptions=Index vector (dialog),Index vector (dialog)  Indices=-1,hres+1:hres*2  OutputSizes=1,1
  Selector2 : Selector  NumberOfDimensions=2  InputPortWidth=3  IndexOptions=Index vector (dialog),Index vector (dialog)  Indices=-1,hres*2+1:hres*3  OutputSizes=1,1
  R : Outport
  G : Outport  Port=2
  B : Outport  Port=3
  wires:
  In1/1 -> Selector1/1, Selector/1, Selector2/1
  Selector/1 -> R/1
  Selector1/1 -> G/1
  Selector2/1 -> B/1

== system FishEyeTestNonCardboard_cs_old/BMW_X5_SUV_1/right_fish_CM_Demux ==
  In1 : Inport
  Selector : Selector  NumberOfDimensions=2  InputPortWidth=3  IndexOptions=Index vector (dialog),Index vector (dialog)  Indices=-1,1:hres  OutputSizes=1,1
  Selector1 : Selector  NumberOfDimensions=2  InputPortWidth=3  IndexOptions=Index vector (dialog),Index vector (dialog)  Indices=-1,hres+1:hres*2  OutputSizes=1,1
  Selector2 : Selector  NumberOfDimensions=2  InputPortWidth=3  IndexOptions=Index vector (dialog),Index vector (dialog)  Indices=-1,hres*2+1:hres*3  OutputSizes=1,1
  R : Outport
  G : Outport  Port=2
  B : Outport  Port=3
  wires:
  In1/1 -> Selector1/1, Selector/1, Selector2/1
  Selector/1 -> R/1
  Selector1/1 -> G/1
  Selector2/1 -> B/1

== system FishEyeTestNonCardboard_cs_old/BMW_X5_SUV_1/SELF_Demux/compas converter ==
  rotz [rad] : Inport
  cart2compas : Subsystem
  rad2deg : Gain  Gain=180/pi
  heading [deg] : Outport
  wires:
  rad2deg/1 -> cart2compas/1(Angle [deg])
  rotz [rad]/1 -> rad2deg/1
  cart2compas/1(heading [deg]) -> heading [deg]/1

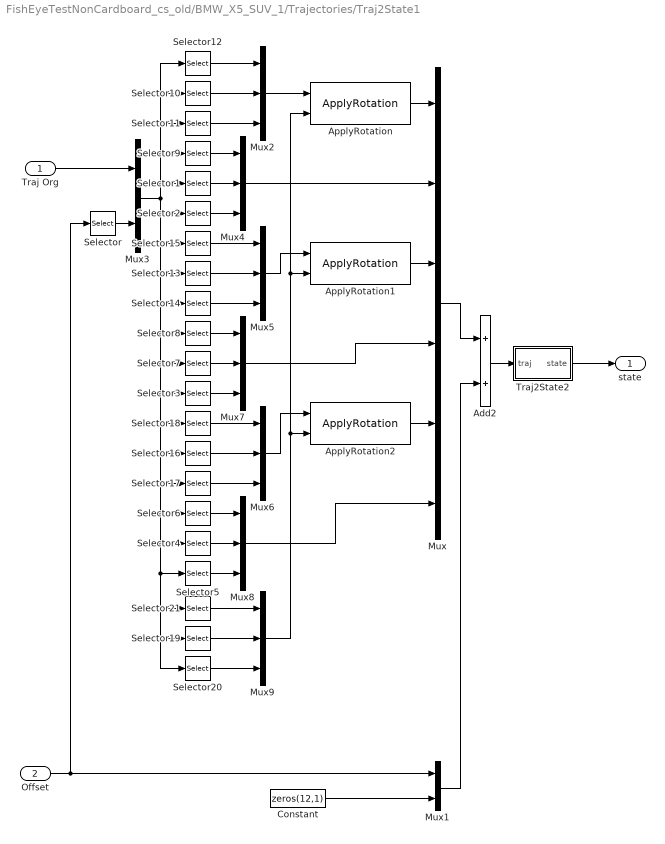
== system FishEyeTestNonCardboard_cs_old/BMW_X5_SUV_1/Trajectories/Traj2State1 ==
  Traj Org : Inport
  Offset : Inport  Port=2
  Add2 : Sum
  ApplyRotation : PreScanSimulinkLibrary/ApplyRotation  SystemSampleTime=-1
  ApplyRotation1 : PreScanSimulinkLibrary/ApplyRotation  SystemSampleTime=-1
  ApplyRotation2 : PreScanSimulinkLibrary/ApplyRotation  SystemSampleTime=-1
  Constant : Constant  Value=zeros(12,1)
  Mux : Mux  Inputs=6
  Mux1 : Mux  Inputs=2
  Mux{2,4..9} (7 alike) : Mux  Inputs=3
  Mux3 : Mux  Inputs=2
  Selector : Selector  InputPortWidth=6  IndexOptions=Index vector (dialog)  Indices=[4 5 6]  OutputSizes=1
  Selector1 : Selector  InputPortWidth=21  IndexOptions=Index vector (dialog)  Indices=[5]  OutputSizes=1
  Selector10 : Selector  InputPortWidth=21  IndexOptions=Index vector (dialog)  Indices=[2]  OutputSizes=1
  Selector11 : Selector  InputPortWidth=21  IndexOptions=Index vector (dialog)  Indices=[3]  OutputSizes=1
  Selector12 : Selector  InputPortWidth=21  IndexOptions=Index vector (dialog)  Indices=[1]  OutputSizes=1
  Selector13 : Selector  InputPortWidth=21  IndexOptions=Index vector (dialog)  Indices=[8]  OutputSizes=1
  Selector14 : Selector  InputPortWidth=21  IndexOptions=Index vector (dialog)  Indices=[9]  OutputSizes=1
  Selector15 : Selector  InputPortWidth=21  IndexOptions=Index vector (dialog)  Indices=[7]  OutputSizes=1
  Selector16 : Selector  InputPortWidth=21  IndexOptions=Index vector (dialog)  Indices=[14]  OutputSizes=1
  Selector17 : Selector  InputPortWidth=21  IndexOptions=Index vector (dialog)  Indices=[15]  OutputSizes=1
  Selector18 : Selector  InputPortWidth=21  IndexOptions=Index vector (dialog)  Indices=[13]  OutputSizes=1
  Selector19 : Selector  InputPortWidth=21  IndexOptions=Index vector (dialog)  Indices=[20]  OutputSizes=1
  Selector2 : Selector  InputPortWidth=21  IndexOptions=Index vector (dialog)  Indices=[6]  OutputSizes=1
  Selector20 : Selector  InputPortWidth=21  IndexOptions=Index vector (dialog)  Indices=[21]  OutputSizes=1
  Selector21 : Selector  InputPortWidth=21  IndexOptions=Index vector (dialog)  Indices=[19]  OutputSizes=1
  Selector3 : Selector  InputPortWidth=21  IndexOptions=Index vector (dialog)  Indices=[12]  OutputSizes=1
  Selector4 : Selector  InputPortWidth=21  IndexOptions=Index vector (dialog)  Indices=[17]  OutputSizes=1
  Selector5 : Selector  InputPortWidth=21  IndexOptions=Index vector (dialog)  Indices=[18]  OutputSizes=1
  Selector6 : Selector  InputPortWidth=21  IndexOptions=Index vector (dialog)  Indices=[16]  OutputSizes=1
  Selector7 : Selector  InputPortWidth=21  IndexOptions=Index vector (dialog)  Indices=[11]  OutputSizes=1
  Selector8 : Selector  InputPortWidth=21  IndexOptions=Index vector (dialog)  Indices=[10]  OutputSizes=1
  Selector9 : Selector  InputPortWidth=21  IndexOptions=Index vector (dialog)  Indices=[4]  OutputSizes=1
  Traj2State2 : Subsystem
  state : Outport
  wires:
  Mux9/1 -> ApplyRotation2/2, ApplyRotation1/2, ApplyRotation/2
  Selector20/1 -> Mux9/3
  Selector19/1 -> Mux9/2
  Selector21/1 -> Mux9/1
  Selector5/1 -> Mux8/3
  Selector4/1 -> Mux8/2
  Selector6/1 -> Mux8/1
  Mux8/1 -> Mux/6
  Mux6/1 -> ApplyRotation2/1
  Mux7/1 -> Mux/4
  ApplyRotation2/1 -> Mux/5
  Selector3/1 -> Mux7/3
  Selector7/1 -> Mux7/2
  Selector8/1 -> Mux7/1
  Mux4/1 -> Mux/2
  Mux5/1 -> ApplyRotation1/1
  ApplyRotation1/1 -> Mux/3
  Mux2/1 -> ApplyRotation/1
  ApplyRotation/1 -> Mux/1
  Selector2/1 -> Mux4/3
  Selector1/1 -> Mux4/2
  Selector9/1 -> Mux4/1
  Selector17/1 -> Mux6/3
  Selector16/1 -> Mux6/2
  Selector18/1 -> Mux6/1
  Selector14/1 -> Mux5/3
  Selector13/1 -> Mux5/2
  Selector15/1 -> Mux5/1
  Selector11/1 -> Mux2/3
  Selector10/1 -> Mux2/2
  Selector12/1 -> Mux2/1
  Mux3/1 -> Selector8/1, Selector7/1, Selector3/1, Selector18/1, Selector16/1, Selector17/1, Selector6/1, Selector20/1, Selector19/1, Selector21/1, Selector5/1, Selector4/1, Selector14/1, Selector13/1, Selector15/1, Selector2/1, Selector1/1, Selector9/1, Selector12/1, Selector10/1, Selector11/1
  Mux1/1 -> Add2/2
  Constant/1 -> Mux1/2
  Add2/1 -> Traj2State2/1(traj)
  Selector/1 -> Mux3/2
  Traj Org/1 -> Mux3/1
  Offset/1 -> Mux1/1, Selector/1
  Mux/1 -> Add2/1
  Traj2State2/1(state) -> state/1
